simulink model "AverageMaxMin"  (R2021a)
settings: Solver=FixedStepDiscrete  StartTime=0.0  StopTime=10.0  RelTol=1e-3
settings Model: SimulationMode=accelerator  Creator=hp  LastModifiedBy=hp
settings OptimizationCC: DefaultParameterBehavior=Inlined  EnhancedBackFolding=on  PassReuseOutputArgsAs=Individual arguments  ZeroExternalMemoryAtStartup=off  ZeroInternalMemoryAtStartup=off  OptimizeBlockOrder=speed  DifferentSizesBufferReuse=on  OptimizationCustomize=off  EfficientTunableParamExpr=on
settings DebuggingCC: ParameterTunabilityLossMsg=error
settings SFSimCC: MATLABDynamicMemAlloc=off
settings RTWCC: SystemTargetFile=ert.tlc  GenCodeOnly=on  TemplateMakefile=ert_default_tmf  GenerateReport=on  IncludeHyperlinkInReport=on  LaunchReport=on  GenerateTraceInfo=on
settings CodeAppCC: ForceParamTrailComments=on  IgnoreCustomStorageClasses=off  OperatorAnnotations=on  SimulinkDataObjDesc=on  SFDataObjDesc=on  InsertBlockDesc=on
settings ERTTargetCC: TargetLangStandard=C99 (ISO)  GenerateSampleERTMain=on  SupportNonFinite=off  SupportComplex=off  InlinedParameterPlacement=NonHierarchical  ERTCustomFileTemplate=example_file_process.tlc  IndentSize=4  EnableUserReplacementTypes=on

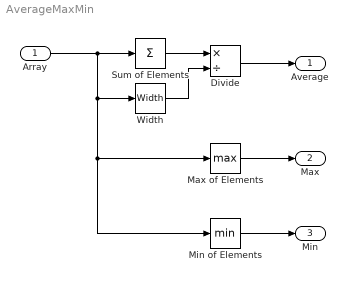
== system AverageMaxMin ==
  Array : Inport  OutDataTypeStr=double  PortDimensions=9
  Divide : Product  Inputs=*/
  Max of Elements : MinMax  Function=max
  Min of Elements : MinMax
  Sum of Elements : Sum  Inputs=+
  Width : Width
  Average : Outport
  Max : Outport  Port=2
  Min : Outport  Port=3
  wires:
  Sum of Elements/1 -> Divide/1
  Array/1 -> Width/1, Min of Elements/1, Max of Elements/1, Sum of Elements/1
  Divide/1 -> Average/1
  Max of Elements/1 -> Max/1
  Min of Elements/1 -> Min/1
  Width/1 -> Divide/2
